simulink model "Bike2ndOrder"  (R2018a)
settings: Solver=VariableStepAuto  StartTime=0.0  StopTime=2  RelTol=1e-3
values from neighbouring files (symbols this model uses):
  A = [0, 1; (m*g*h)/J, 0]    [lqrBike.m]    (also in secondOrderBike.m; setBikeStateSpace.m = Bike.A)
  B = [0; 1]    [lqrBike.m]    (also in plotBikeGains.m = B(:,2); secondOrderBike.m; setBikeStateSpace.m = Bike.B)
  b = 1.08    [secondOrderBike.m]
  C = eye(4)    [getBikeSymbolicStateSpace.m]    (also in lqrBike.m = [(m*h*V^2)/(b*J), (V*D)/(J*b)]; secondOrderBike.m = [(m*h*V^2)/(b*J), (V*D)/(J*b)]; setBikeStateSpace.m = Bike.C)
  D = m * a * h    (= 3.9325)    [secondOrderBike.m]    (also in setBikeStateSpace.m = Bike.D)
  g = 9.81    [secondOrderBike.m]
  h = -uu(3)    [plotBikeStateVariables.m]    (also in secondOrderBike.m = 0.55)
  J = m * h * h    (= 8.31875)    [secondOrderBike.m]
  K = lqr(A, B, Q, R)    [lqrBike.m]    (also in plotBikeGains.m = zeros(N, 4); plotKpKd.m = Kp + Kd * s; secondOrderBike.m = 1)
  m = 27.5    [secondOrderBike.m]
  V = size*V    [drawBike.m]    (also in secondOrderBike.m = 3)
undefined symbols (not defined in the file or in its folder): Continuous, Time
libraries: simulink_extras x4, simulink x2, dspsrcs4 x2, ctrlSharedLib x1
settings Model: Creator=Philip  LastModifiedBy=Philip

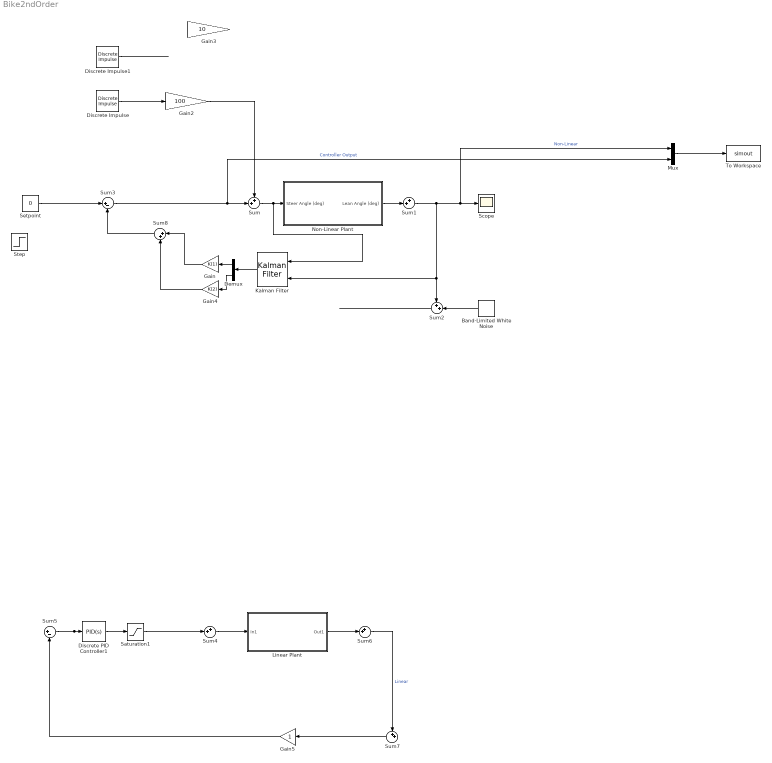
== system Bike2ndOrder ==
  Band-Limited White Noise : simulink/Sources/Band-Limited White Noise  Cov=1e-9  Ts=0.001  seed=[23341]
  Demux : Demux  Outputs=2
  Discrete Impulse : dspsrcs4/Discrete  Impulse  Delay=0  SampleTime=0.001  FrameSample=1  OutputFrames=off  dataType=double  isSigned=on  wordLen=16  udDataType=sfix(16)  fracBitsMode=Best precision  numFracBits=15  OutDataTypeStr=double  LastOutDataTypeStr=double
  Discrete Impulse1 : dspsrcs4/Discrete  Impulse  Delay=0  SampleTime=0.001  FrameSample=1  OutputFrames=off  dataType=double  isSigned=on  wordLen=16  udDataType=sfix(16)  fracBitsMode=Best precision  numFracBits=15  OutDataTypeStr=double  LastOutDataTypeStr=double
  Discrete PID Controller1 : simulink/Continuous/PID Controller  Controller=PID  TimeDomain=Continuous-time  SampleTime=-1  IntegratorMethod=Trapezoidal  FilterMethod=Trapezoidal  Form=Parallel  UseFilter=on  ControllerParametersSource=internal  P=11.5796502347613  I=37.2822131654474  D=0.440837613798774  N=1162.80366349051  InitialConditionSource=internal  InitialConditionForIntegrator=0  InitialConditionForFilter=0  ExternalReset=none  LimitOutput=on  UpperSaturationLimit=45  LowerSaturationLimit=-45  LinearizeAsGain=off  AntiWindupMode=clamping  Kb=1  TrackingMode=off  Kt=1  PParamMin=[]  PParamMax=[]  IParamMin=[]  IParamMax=[]  DParamMin=[]  DParamMax=[]  NParamMin=[]  NParamMax=[]  KbParamMin=[]  KbParamMax=[]  KtParamMin=[]  KtParamMax=[]  POutMin=[]  POutMax=[]  IOutMin=[]  IOutMax=[]  DOutMin=[]  DOutMax=[]  NOutMin=[]  NOutMax=[]  KbOutMin=[]  KbOutMax=[]  KtOutMin=[]  KtOutMax=[]  IntegratorOutMin=[]  IntegratorOutMax=[]  FilterOutMin=[]  FilterOutMax=[]  SumOutMin=[]  SumOutMax=[]  SumI1OutMin=[]  SumI1OutMax=[]  SumI2OutMin=[]  SumI2OutMax=[]  SumI3OutMin=[]  SumI3OutMax=[]  SumDOutMin=[]  SumDOutMax=[]  SaturationOutMin=[]  SaturationOutMax=[]  IntegratorContinuousStateAttributes=''  IntegratorStateMustResolveToSignalObject=off  IntegratorRTWStateStorageClass=Auto  FilterContinuousStateAttributes=''  FilterStateMustResolveToSignalObject=off  FilterRTWStateStorageClass=Auto  DifferentiatorICPrevScaledInput=0  DifferentiatorOutMin=[]  DifferentiatorOutMax=[]  FilterDiffOutCoefMin=[]  FilterDiffOutCoefMax=[]  SumDenOutMin=[]  SumDenOutMax=[]  SumNumOutMin=[]  SumNumOutMax=[]  ReciprocalOutMin=[]  ReciprocalOutMax=[]  DivideOutMin=[]  DivideOutMax=[]  TunerSelectOption=Transfer Function Based (PID Tuner App)
  Gain : Gain  Gain=K(1)
  Gain2 : Gain  Gain=100
  Gain3 : Gain  Gain=10
  Gain4 : Gain  Gain=K(2)
  Gain5 : Gain
  Kalman Filter : ctrlSharedLib/Kalman Filter  TimeDomain=Continuous-Time  UseCurrentEstimator=on  ModelSource=Individual A, B, C, D matrices  ModelSourceVariable=Gss  A=A  B=B  C=C  D=0  NumberOfStates=1  NumberOfInputs=1  NumberOfOutputs=1  InitialEstimateSource=Dialog  X0=0  P0=10  UseK=off  UseGH=off  NumberOfProcessNoiseInputs=1  G=1  TimeInvariantG=on  H=0  TimeInvariantH=on  Q=0.01  TimeInvariantQ=on  R=0.001  TimeInvariantR=on  N=0  TimeInvariantN=on  AddInputPort=on  AddEnablePort=off  OutputEstimatedY=off  OutputP=off  Ts=-1
      settings: SourceProductBaseCode=CT
  Linear Plant : Subsystem
  Mux : Mux  Inputs=2
  Non-Linear Plant : Subsystem
  Saturation1 : Saturate  UpperLimit=45  LowerLimit=-45
  Scope : Scope
  Setpoint : Constant  Value=0
  Step : Step  Time=0  SampleTime=0
  Sum{,1..2,4,6..7} (6 alike) : Sum  Inputs=++|
  Sum3 : Sum  Inputs=|+-
  Sum5 : Sum  Inputs=|+-
  Sum8 : Sum  Inputs=|++
  To Workspace : ToWorkspace  VariableName=simout  SaveFormat=Structure With Time  SampleTime=0.01
  wires:
  Sum/1 -> Kalman Filter/1, Non-Linear Plant/1(Steer Angle (deg))
  Sum3/1 -> Mux/2, Sum/2  "Controller Output"
  Sum1/1 -> Scope/1, Mux/1, Sum2/1, Kalman Filter/2  "Non-Linear"
  Sum2/1 -> ?
  Band-Limited White Noise/1 -> Sum2/2
  Setpoint/1 -> Sum3/1
  Discrete Impulse/1 -> Gain2/1
  Gain2/1 -> Sum/1
  Discrete Impulse1/1 -> ?
  Mux/1 -> To Workspace/1
  ? -> Sum1/1
  Non-Linear Plant/1(Lean Angle (deg)) -> Sum1/2
  Saturation1/1 -> Sum4/2
  Sum5/1 -> Discrete PID Controller1/1
  Discrete PID Controller1/1 -> Saturation1/1
  ? -> Sum7/2
  Gain5/1 -> Sum5/2
  Sum7/1 -> Gain5/1
  Linear Plant/1(Out1) -> Sum6/2
  Sum4/1 -> Linear Plant/1(In1)
  Sum6/1 -> Sum7/1  "Linear"
  Kalman Filter/1 -> Demux/1
  Demux/1 -> Gain/1
  Demux/2 -> Gain4/1
  Gain/1 -> Sum8/1
  Gain4/1 -> Sum8/2
  Sum8/1 -> Sum3/2

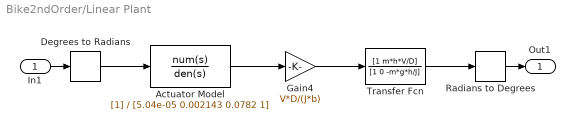
== system Bike2ndOrder/Linear Plant ==
  In1 : Inport
  Actuator Model : TransferFcn  Denominator=[5.04e-05 0.002143 0.0782 1]
  Degrees to Radians : simulink_extras/Transformations/Degrees to Radians
  Gain4 : Gain  Gain=V*D/(J*b)
  Radians to Degrees : simulink_extras/Transformations/Radians to Degrees
  Transfer Fcn : TransferFcn  Numerator=[1 m*h*V/D]  Denominator=[1 0 -m*g*h/J]
  Out1 : Outport
  wires:
  Transfer Fcn/1 -> Radians to Degrees/1
  Gain4/1 -> Transfer Fcn/1
  In1/1 -> Degrees to Radians/1
  Degrees to Radians/1 -> Actuator Model/1
  Actuator Model/1 -> Gain4/1
  Radians to Degrees/1 -> Out1/1

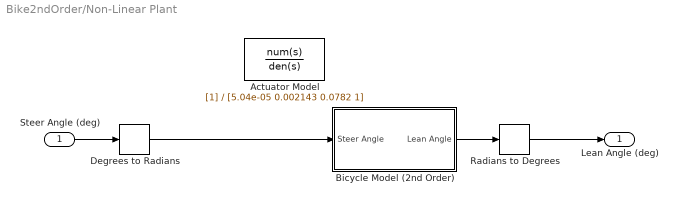
== system Bike2ndOrder/Non-Linear Plant ==
  Steer Angle (deg) : Inport
  Actuator Model : TransferFcn  Denominator=[5.04e-05 0.002143 0.0782 1]
  Bicycle Model (2nd Order) : Subsystem
  Degrees to Radians : simulink_extras/Transformations/Degrees to Radians
  Radians to Degrees : simulink_extras/Transformations/Radians to Degrees
  Lean Angle (deg) : Outport
  wires:
  Bicycle Model (2nd Order)/1(Lean Angle) -> Radians to Degrees/1
  Degrees to Radians/1 -> Bicycle Model (2nd Order)/1(Steer Angle)
  Radians to Degrees/1 -> Lean Angle (deg)/1
  Steer Angle (deg)/1 -> Degrees to Radians/1

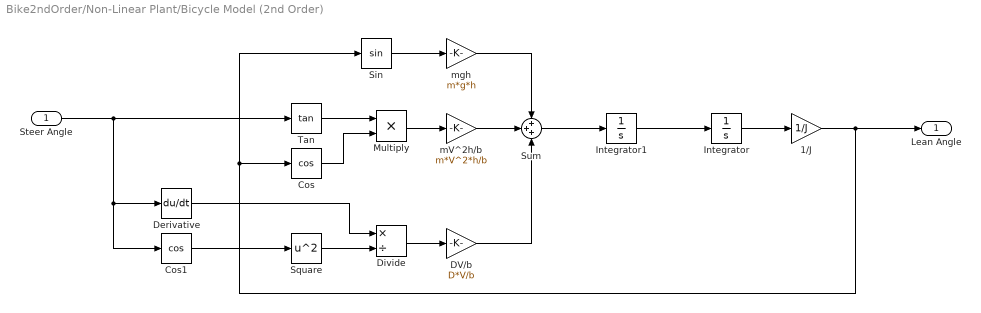
== system Bike2ndOrder/Non-Linear Plant/Bicycle Model (2nd Order) ==
  Steer Angle : Inport
  1/J : Gain  Gain=1/J
  Cos : Trigonometry  Operator=cos
  Cos1 : Trigonometry  Operator=cos
  DV/b : Gain  Gain=D*V/b
  Derivative : Derivative  CoefficientInTFapproximation=0.00000001
  Divide : Product  Inputs=*/
  Integrator : Integrator
  Integrator1 : Integrator
  Multiply : Product
  Sin : Trigonometry
  Square : Math  Operator=square  SaturateOnIntegerOverflow=on
  Sum : Sum  Inputs=+++
  Tan : Trigonometry  Operator=tan
  mV^2h/b : Gain  Gain=m*V^2*h/b
  mgh : Gain  Gain=m*g*h
  Lean Angle : Outport
  wires:
  DV/b/1 -> Sum/3
  1/J/1 -> Cos/1, Sin/1, Lean Angle/1
  Sin/1 -> mgh/1
  Integrator1/1 -> Integrator/1
  Steer Angle/1 -> Derivative/1, Cos1/1, Tan/1
  mgh/1 -> Sum/1
  Tan/1 -> Multiply/1
  Sum/1 -> Integrator1/1
  Cos/1 -> Multiply/2
  Divide/1 -> DV/b/1
  Cos1/1 -> Square/1
  Derivative/1 -> Divide/1
  Square/1 -> Divide/2
  Integrator/1 -> 1/J/1
  mV^2h/b/1 -> Sum/2
  Multiply/1 -> mV^2h/b/1
